simulink model "Sub1"  (R2024a)
settings: Solver=FixedStepDiscrete  StartTime=0.0  StopTime=1  FixedStep=7.5e-05  RelTol=1e-3  EnableMultiTasking=on
undefined symbols (not defined in the file or in its folder): D1, D11, Delta
libraries: spsSeriesRLCBranchLib x41, spsLoadFlowBusLib x29, spsDistributedParametersLineLib x19, spsThreePhaseSeriesRLCLoadLib x15, spsThreePhaseTransformerTwoWindingsLib x13, spsThreePhaseParallelRLCLoadLib x11, spsThreePhaseVIMeasurementLib x11, spsSynchronousMachinepuStandardLib x7, spsExcitationSystemLib x7, spsHydraulicTurbineandGovernorLib x7, spsGenericPowerSystemStabilizerLib x7, spsMultiBandPowerSystemStabilizerLib x7
(part 1 of 5)
settings Model: Creator=The MathWorks, Inc.  LastModifiedBy=dilu2
settings SolverCC: AlgebraicLoopSolver=TrustRegion
settings DataIOCC: SaveFormat=StructureWithTime  SaveOutput=off  SignalLogging=off  DSMLogging=off  SaveTime=off  ReturnWorkspaceOutputs=off
settings OptimizationCC: ExpressionDepthLimit=2147483647  LifeSpan=inf
settings DebuggingCC: UnderspecifiedInitializationDetection=Classic  MergeDetectMultiDrivingBlocksExec=none  SolverPrmCheckMsg=warning  FcnCallInpInsideContextMsg=warning  UnconnectedInputMsg=warning  UnconnectedOutputMsg=warning  UnconnectedLineMsg=warning  StateNameClashWarn=warning  SFUnexpectedBacktrackingDiag=warning  SFNoUnconditionalDefaultTransitionDiag=warning  SFExecutionAtInitializationDiag=none  ArithmeticOperatorsInVariantConditions=warning
settings HardwareCC: ProdBitPerPointer=32  ProdBitPerSizeT=32  ProdBitPerPtrDiffT=32  ProdLargestAtomicFloat=None  ProdIntDivRoundTo=Undefined  ProdEndianess=Unspecified  ProdWordSize=32  ProdHWDeviceType=32-bit Generic
settings ModelReferenceCC: EnableRefExpFcnMdlSchedulingChecks=on  PropagateSignalLabelsOutOfModel=off
settings SFSimCC: SimUseLocalCustomCode=off  CustomCodeUndefinedFunction=UseInterfaceOnly
settings RTWCC: RTWUseLocalCustomCode=off  GPUComputeCapability=3.5
settings CodeAppCC: StateflowObjectComments=on
settings GRTTargetCC: TargetLangStandard=C89/C90 (ANSI)  CombineOutputUpdateFcns=off  GRTInterface=on
settings ConfigComp: CovMetricSettings=dw  CovSaveCumulativeToWorkspaceVar=on  CovSaveSingleToWorkspaceVar=on  CovExternalEMLEnable=off  CovSFcnEnable=off
settings SimscapeCC: SimscapeNormalizeSystem=off

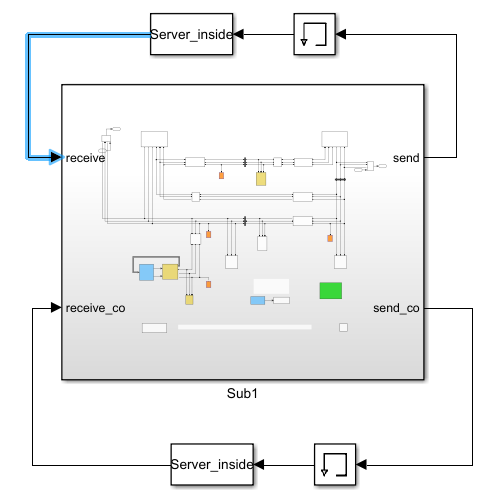
[thumbnail: Simulink's stored preview of the top-level diagram]
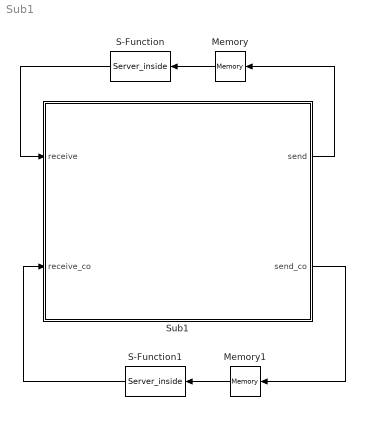
== system Sub1 ==
  Memory : Memory
  Memory1 : Memory
  S-Function : S-Function  FunctionName=Server_inside  SFunctionDeploymentMode=off  EnableBusSupport=off
  S-Function1 : S-Function  FunctionName=Server_inside  SFunctionDeploymentMode=off  EnableBusSupport=off
  Sub1 : Subsystem
  wires:
  Memory/1 -> S-Function/1
  Sub1/1(send) -> Memory/1
  S-Function/1 -> Sub1/1(receive)
  Memory1/1 -> S-Function1/1
  S-Function1/1 -> Sub1/2(receive_co)
  Sub1/2(send_co) -> Memory1/1

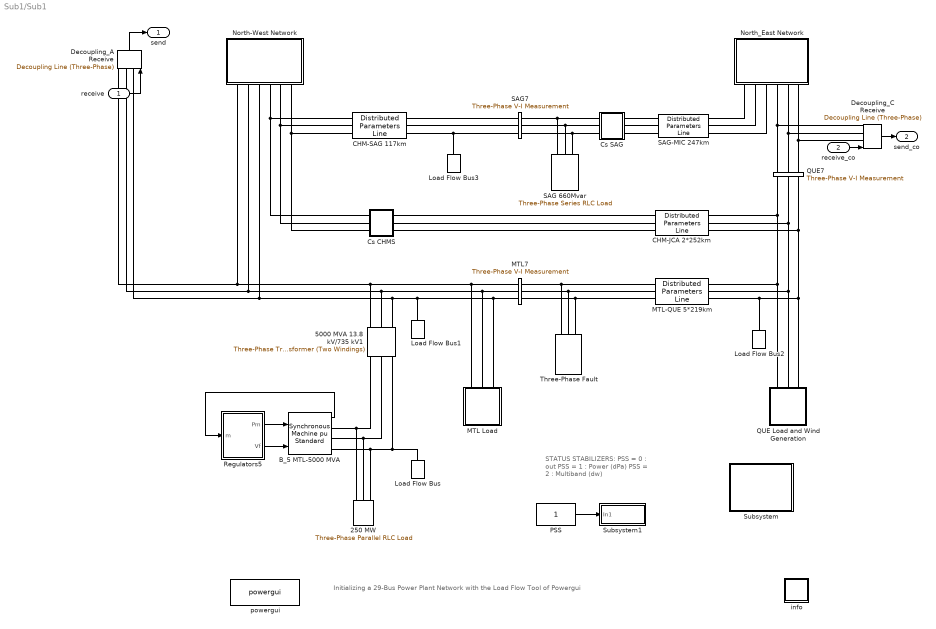
== system Sub1/Sub1 ==
  note: STATUS STABILIZERS:
      | PSS = 0 :  out
      | PSS = 1 :  Power (dPa)
      | PSS = 2 :  Multiband (dw)
  note: Initializing a 29-Bus Power Plant Network with the Load Flow Tool of Powergui
  receive : Inport
  receive_co : Inport  Port=2
  250 MW : spsThreePhaseParallelRLCLoadLib/Three-Phase Parallel RLC Load  LConnTagsString=A|B|C  Configuration=Y (grounded)  NominalVoltage=(13800)*1  Vabc=[1e3 1e3 1e3]  Vabcp=[1e3 1e3 1e3]  NominalFrequency=60  UnbalancedPower=off  ActivePower=250000000  InductivePower=0  CapacitivePower=0  Pabc=[10e3 9e3 11e3]  QLabc=[100 90 110]  QCabc=[100 90 110]  Pabcp=[10e3 9e3 11e3]  QLabcp=[100 90 110]  QCabcp=[100 90 110]  Measurements=None  LoadType=constant PQ
  5000 MVA 13.8 kV/735 kV1 : spsThreePhaseTransformerTwoWindingsLib/Three-Phase Transformer (Two Windings)  Winding1Connection=Delta (D1)  Winding2Connection=Yg  CoreType=Three single-phase transformers  SetSaturation=off  Hysteresis=off  DataFile='basic_model'  SetInitialFlux=off  Measurements=None  UNITS=pu  NominalPower=[ 5000e6 60 ]  Winding1="[ 13.8e3 0.002  0.0]"  Winding2=[ 735e3 0.002 0.12]  Rm=500  Lm=500  L0=0.5  Saturation="[ 0,0  ;  0.005,1.2  ;  1.0,1.4 ]"  InitialFluxes=[ 0.8 , -0.8 , 0.7 ]  BreakLoop=off  DiscreteSolver=Trapezoidal iterative  DataType=off  TransfoNumber=0
  B_5 MTL-5000 MVA : spsSynchronousMachinepuStandardLib/Synchronous Machine pu Standard  PresetModel=No  MechanicalLoad=Mechanical power Pm  ShowDetailedParameters=on  RotorType=Salient-pole  Units=per unit standard parameters  MeasurementBus=off  NominalParameters="[5000E6  13800   60 ]"  Reactances1=[ 31 32 33 34 35 36 37 ]  Reactances2=[ 1.305, 0.296, 0.252, 0.474, 0.243, 0.18 ]  dAxisTimeConstants=Short-circuit  qAxisTimeConstants=Open-circuit  TimeConstants1=[]  TimeConstants2=[]  TimeConstants3=[]  TimeConstants4=[]  TimeConstants5=[ 1.01, 0.053, 0.1 ]  TimeConstants6=[]  TimeConstants7=[]  TimeConstants8=[]  StatorResistance=2.8544e-3  Mechanical="[ 3.7 0  32]"  PolePairs=32  InitialConditions=[0 -113.876 0.904539 0.904539 0.904539 -42.1129 -162.113 77.8871 1.28555]  SetSaturation=off  Saturation=[0.6404,0.7127,0.8441,0.9214,0.9956,1.082,1.19,1.316,1.457;0.7,0.7698,0.8872,0.9466,0.9969,1.046,1.1,1.151,1.201]  LoadFlowParameters=[1 4000000000 0 0 0]  TsPowergui=0  TsBlock=-1  IterativeModel=Trapezoidal non iterative  IterativeDiscreteModel=Trapezoidal non iterative  BusType=PV  Pref=4500000000  Qref=0  Qmin=-Inf  Qmax=Inf  PLF=0  QLF=0
  CHM-JCA 2*252km : spsDistributedParametersLineLib/Distributed Parameters Line  Phases=3  Length=252  Frequency=60  Resistance="[0.01273  0.3864]/2"  Inductance="[0.9337e-3  4.1264e-3]/2"  Capacitance=[12.74e-9 7.751e-9]*2  x1=[-0.0015 2.14221721230477e-08 15714.2625948139 -742648.807936558;-0.001425 2.14666224013432e-08 36703.0761534274 -741907.71197206;-0.00135 2.14939125901414e-08 57662.5498345396 -740573.546334181;-0.001275 2.1504020874083e-08 78575.9289555807 -738647.377534517;-0.0012 2.14969391727604e-08 99426.4956812668 -736130.745322936;-0.001125 2.14726731471772e-08 120197.582387582 -733025.661456722;-0.00105 2.14312421952232e-08 140872.584985621 -729334.608092408;-0.000975 2.13726794361672e-08 161434.976194645 -725060.535801579;-0.0009 2.1297031684183e-08 181868.318753737 -720206.861212228;-0.000825 2.12043594109259e-08 202156.278561496 -714777.464277558;-0.00075 2.10947366971934e-08 222282.637733268 -708776.685174407;-0.000675 2.09682511737053e-08 242231.307565474 -702209.320833775;-0.0006 2.08250039510541e-08 261986.341396676 -695080.621106231;-0.000525 2.06651095388776e-08 281531.94735509 -687396.284565265;-0.00045 2.04886957543225e-08 300852.500982373 -679162.453951933;-0.000375 2.02959036198689e-08 319932.557723567 -670385.711264446;-0.0003 2.00868872505994e-08 338756.86527325 -661073.072496619;-0.000225 1.98618137310014e-08 357310.375767987 -651231.982029396;-0.00015 1.96208629814028e-08 375578.257815367 -640870.306679922;-7.5e-05 1.93642276141461e-08 393545.908349989 -629996.329412933]  x2=[-0.0015 1.38205484326445e-08 -209700.603633361 -700128.672634782;-0.001425 1.37920737733266e-08 -189823.746323616 -705777.196573591;-0.00135 1.37525739412601e-08 -169795.146815461 -710861.533020212;-0.001275 1.37020805120064e-08 -149630.815664894 -715377.617633884;-0.0012 1.36406338492402e-08 -129346.871929713 -719321.840325663;-0.001125 1.35682830724837e-08 -108959.530284185 -722691.048144279;-0.00105 1.34850860178407e-08 -88485.088057284 -725482.547796553;-0.000975 1.33911091917638e-08 -67939.9122048576 -727694.107800373;-0.0009 1.32864277178898e-08 -47340.4262261302 -729323.960268511;-0.000825 1.31711252769873e-08 -26703.0970350105 -730370.802321841;-0.00075 1.30452940400633e-08 -6044.42179669201 -730833.797130843;-0.000675 1.29090345946834e-08 14619.085259928 -730712.57458455;-0.0006 1.27624558645634e-08 35270.9060434707 -730007.231586412;-0.000525 1.26056750224974e-08 55894.5318043853 -728718.33197683;-0.00045 1.24388173966917e-08 76473.4763317904 -726846.906082429;-0.000375 1.22620163705793e-08 96991.2891322993 -724394.449892436;-0.0003 1.20754132761955e-08 117431.568580292 -721362.923862806;-0.000225 1.18791572811987e-08 137777.975029126 -717754.751349063;-0.00015 1.16734052696285e-08 158014.243872794 -713572.816669108;-7.5e-05 1.14583217164948e-08 178124.19854761 -708820.462797537]  x3=[-0.0015 5.44608144766307e-11 0.894999887860962 -284.908126309021;-0.001425 5.3877879205201e-11 8.94952227176843 -284.768519994184;-0.00135 5.32518747814939e-11 16.9968905445041 -284.401274081569;-0.001275 5.25833016238674e-11 25.0306717629996 -283.806682141938;-0.0012 5.18726941794743e-11 33.0444438454699 -282.98521948299;-0.001125 5.11206204970331e-11 41.0318007051272 -281.937542769407;-0.00105 5.03276817727381e-11 48.9863573711083 -280.664489497923;-0.000975 4.94945118696735e-11 56.9017550925234 -279.167077327845;-0.0009 4.86217768111116e-11 64.7716664215435 -277.446503267551;-0.000825 4.7710174248105e-11 72.589800271466 -275.504142717618;-0.00075 4.67604329017947e-11 80.3499069457126 -273.341548371352;-0.000675 4.57733119808813e-11 88.0457831337417 -270.960448973583;-0.0006 4.47496005747255e-11 95.6712768698793 -268.36274793874;-0.000525 4.36901170225622e-11 103.220292451107 -265.550521829281;-0.00045 4.25957082593322e-11 110.686795309872 -262.526018695731;-0.000375 4.14672491386559e-11 118.064816838032 -259.291656279619;-0.0003 4.03056417334883e-11 125.348459158063 -255.850020080773;-0.000225 3.9111814615016e-11 132.53189983774 -252.20386129051;-0.00015 3.78867221103713e-11 139.609396544492 -248.35609459238;-7.5e-05 3.66313435397578e-11 146.575291635741 -244.309795832209]  x4=[-0.0015 3.11331321468092e-11 -3172.83341993578 -10043.3125795458;-0.001425 3.24270107310813e-11 -2887.6355082528 -10128.9965094917;-0.00135 3.3694967659125e-11 -2600.12926492682 -10206.5834746068;-0.001275 3.49359893455722e-11 -2310.54451804977 -10276.0114530582;-0.0012 3.61490837366751e-11 -2019.11275723751 -10337.2249451823;-0.001125 3.73332811033385e-11 -1726.06694858057 -10390.17501785;-0.00105 3.84876348163062e-11 -1431.64134841465 -10434.8193435835;-0.000975 3.96112221028823e-11 -1136.07131605966 -10471.1222343919;-0.0009 4.07031447845814e-11 -839.593125677075 -10499.0546702996;-0.000825 4.17625299951187e-11 -542.443777396034 -10518.5943225447;-0.00075 4.2788530878166e-11 -244.860807859011 -10529.7255714284;-0.000675 4.37803272643159e-11 52.9178996613191 -10532.4395188004;-0.0006 4.4737126326712e-11 350.65430542233 -10526.7339951728;-0.000525 4.56581632148236e-11 648.110403496778 -10512.613561454;-0.00045 4.65427016658546e-11 945.048412031093 -10490.0895053025;-0.000375 4.73900345933011e-11 1241.23096332455 -10459.1798321041;-0.0003 4.81994846521856e-11 1536.42129357741 -10419.9092505789;-0.000225 4.8970404780516e-11 1830.38343215621 -10372.3091530287;-0.00015 4.97021787165371e-11 2122.88239022515 -10316.4175902431;-7.5e-05 5.03942214913611e-11 2413.68434859253 -10252.2792410825]  x5=0.00142516474882927  V1=ones(3,3)  V2=ones(3,3)  I1=ones(3,3)  I2=ones(3,3)  nHarmo=1  Measurements=None  Decoupling=on  VsMag0=[606505.937088368 606505.596193701 606505.952336057]  VrMag0=[596743.7373363 596743.911083318 596743.706580261]  VsAngle0=[3.61218308623452 -116.387796657607 123.612221103661]  VrAngle0=[-14.2738568821649 -134.273869923457 105.726122150019]  IsMag0=[234.023435046449 234.012623108521 234.010085804401]  IrMag0=[8650.90032066112 8650.90619032951 8650.91364627791]  IsAngle0=[2.58186505637036 -117.420380634471 122.583034804929]  IrAngle0=[-15.1321830152081 -135.132103549671 104.86782305054]
      settings: AttributesFormatString=\n  LibrarySourceBlock=sps_lib/Power Grid Elements/Distributed Parameters Line
  CHM-SAG 117km : spsDistributedParametersLineLib/Distributed Parameters Line  Phases=3  Length=117  Frequency=60  Resistance="[0.01273  0.3864]"  Inductance="[0.9337e-3  4.1264e-3]"  Capacitance=[12.74e-9 7.751e-9]  x1=[-0.000675 1.99891011372801e-08 161384.253868444 -730188.013920946;-0.0006 1.9861149341103e-08 181962.578167346 -725333.731757044;-0.000525 1.97173208460285e-08 202395.444365381 -719899.628905954;-0.00045 1.95577306263547e-08 222666.518741945 -713890.04930635;-0.000375 1.93825062560616e-08 242759.596910338 -707309.796924214;-0.0003 1.91917878068296e-08 262658.616771308 -700164.131912621;-0.000225 1.89857277360691e-08 282347.671352842 -692458.766406846;-0.00015 1.87644907650477e-08 301811.021525961 -684199.859958181;-7.5e-05 1.85282537472151e-08 321033.108586336 -675394.014610073]  x2=[-0.000675 1.35443395855415e-08 211241.020698681 -709610.35423456;-0.0006 1.3439585589586e-08 231217.67857916 -703354.834381312;-0.000525 1.33240881945427e-08 251009.504585131 -696537.063435149;-0.00045 1.31979397272621e-08 270600.677433712 -689162.49141785;-0.000375 1.30612410288988e-08 289975.536241081 -681237.013449452;-0.0003 1.29141013743006e-08 309118.593041554 -672766.965035778;-0.000225 1.27566383846562e-08 328014.545168422 -663759.117003934;-0.00015 1.25889779334703e-08 346648.287486673 -654220.670089812;-7.5e-05 1.24112540459421e-08 365004.924467804 -644159.249181932]  x3=[-0.000675 1.53428175208454e-11 931.801693491229 -3923.77003572275;-0.0006 1.4387032050888e-11 1042.3568642952 -3895.8590867212;-0.000525 1.34197458076381e-11 1152.07879097044 -3864.83384757437;-0.00045 1.24417320249186e-11 1260.87976348758 -3830.71911938373;-0.000375 1.14537725119832e-11 1368.67280801389 -3793.54217294102;-0.0003 1.04566570285503e-11 1475.37175643888 -3753.33272692841;-0.000225 9.45118265348109e-12 1580.89131525571 -3710.1229241618;-0.00015 8.43815314760658e-12 1685.14713374358 -3663.94730589641;-7.5e-05 7.41837831121395e-12 1788.05587139634 -3614.84278421495]  x4=[-0.000675 2.95936100054461e-11 34.7429415928699 -1477.32347167436;-0.0006 3.04376849592254e-11 76.4934319413223 -1475.75088744153;-0.000525 3.12574284933605e-11 118.18277461067 -1472.99861052903;-0.00045 3.20521853174128e-11 159.77764377825 -1469.06884106491;-0.000375 3.28213201149371e-11 201.244789142075 -1463.96472044674;-0.0003 3.35642180513446e-11 242.551062500607 -1457.69032883046;-0.000225 3.42802852653917e-11 283.663444250933 -1450.25068186873;-0.00015 3.49689493439035e-11 324.54906978412 -1441.65172670148;-7.5e-05 3.56296597793527e-11 365.175255756689 -1431.90033720193]  x5=0.000661683633385019  V1=ones(3,3)  V2=ones(3,3)  I1=ones(3,3)  I2=ones(3,3)  nHarmo=1  Measurements=None  Decoupling=on  VsMag0=[610584.183721697 610584.009535635 610584.144429957]  VrMag0=[604521.569069116 604521.776249676 604521.565003162]  VsAngle0=[-2.95698942544552 -122.956984245972 117.043027319658]  VrAngle0=[1.15752648646782 -118.842485295545 121.157503589919]  IsMag0=[3301.92473587883 3301.92030404023 3301.91445622762]  IrMag0=[1209.87683704235 1209.87940955581 1209.8866532217]  IsAngle0=[-2.06102029188666 -122.061181862044 117.938965522653]  IrAngle0=[-14.0730509971337 -134.072584557043 105.927076719811]
      settings: AttributesFormatString=\n  LibrarySourceBlock=sps_lib/Power Grid Elements/Distributed Parameters Line
  Cs CHMS : Subsystem  mask{Xc=33/2}
      mask prompts: Xc "Condensator Reactance at  60Hz  (ohm):"
      mask help: Series Compensation
      mask init:
      | Cs=1/Xc/(2*pi*60);
      mask Display: disp('Cs')
  Cs SAG : Subsystem  mask{Xc=22}
      mask prompts: Xc "Condensator Reactance at  60Hz  (ohm):"
      mask help: Series Compensation
      mask init:
      | Cs=1/Xc/(2*pi*60);
      mask Display: disp('Cs')
  Decoupling_A Receive : spsDecouplingLineThreePhaseLib/Decoupling Line (Three-Phase)  Length=252  Frequency=60  Resistance="[0.01273  0.3864]/2"  Inductance="[0.9337e-3  4.1264e-3]/2"  Capacitance=[12.74e-9 7.751e-9]*2  VsMag0=[520613.01336377 520613.032750475 520613.042981105]  VsAngle0=[95.9069967092304 -144.093005822699 -24.0930027089851]  IhsMag0=[3886.8321505435 3886.83229528581 3886.83237166039]  IhsAngle0=[86.4922430478116 -153.507759484046 -33.5077563703122]  ShowPorts=on  ConnectorID=T42_4042_2844522148740_R
      settings: LibrarySourceBlock=|
      | sps_lib/Power Grid Elements/Decoupling Line
      | (Three-Phase)
  Decoupling_C Receive : spsDecouplingLineThreePhaseLib/Decoupling Line (Three-Phase)  Length=252  Frequency=60  Resistance="[0.01273  0.3864]/2"  Inductance="[0.9337e-3  4.1264e-3]/2"  Capacitance=[12.74e-9 7.751e-9]*2  VsMag0=[539326.065002207 539326.156042215 539326.02070903]  VsAngle0=[103.825331452952 -136.17465752961 -16.1746546623784]  IhsMag0=[3629.74540447128 3629.74477875179 3629.75000907213]  IhsAngle0=[47.3040516013799 167.303961970658 -72.6960017677198]  ShowPorts=on  ConnectorID=T42_4044_2849153755848_R
      settings: LibrarySourceBlock=|
      | sps_lib/Power Grid Elements/Decoupling Line
      | (Three-Phase)
  Load Flow Bus : spsLoadFlowBusLib/Load Flow Bus  LConnTagsString=a  Phases=single  Connectors=on one side  ID=MTL_13.8  Vbase=13.8e3  Vref=1  Vangle=0  VLF=1  VLFb=1  VLFc=1  angleLF=-47.86  angleLFb=0  angleLFc=0
      settings: AttributesFormatString=%<ID>\n%<Vbase>V\n%<VLF>pu\n%<angleLF>deg.
  Load Flow Bus1 : spsLoadFlowBusLib/Load Flow Bus  LConnTagsString=a  Phases=single  Connectors=on one side  ID=MTL7  Vbase=735e3  Vref=1  Vangle=0  VLF=1.013  VLFb=1  VLFc=1  angleLF=-23.64  angleLFb=0  angleLFc=0
      settings: AttributesFormatString=%<ID>\n%<Vbase>V\n%<VLF>pu\n%<angleLF>deg.
  Load Flow Bus2 : spsLoadFlowBusLib/Load Flow Bus  LConnTagsString=a  Phases=single  Connectors=on one side  ID=QUE7  Vbase=735e3  Vref=1  Vangle=0  VLF=1.023  VLFb=1  VLFc=1  angleLF=-14.99  angleLFb=0  angleLFc=0
      settings: AttributesFormatString=%<ID>\n%<Vbase>V\n%<VLF>pu\n%<angleLF>deg.
  Load Flow Bus3 : spsLoadFlowBusLib/Load Flow Bus  LConnTagsString=a  Phases=single  Connectors=on one side  ID=SAG7  Vbase=735e3  Vref=1  Vangle=0  VLF=1.036  VLFb=1  VLFc=1  angleLF=-0.1653  angleLFb=0  angleLFc=0
      settings: AttributesFormatString=%<ID>\n%<Vbase>V\n%<VLF>pu\n%<angleLF>deg.
  MTL Load : Subsystem
  MTL-QUE 5*219km : spsDistributedParametersLineLib/Distributed Parameters Line  Phases=3  Length=219  Frequency=60  Resistance="[0.01273  0.3864]/5"  Inductance="[0.9337e-3  4.1264e-3]/5"  Capacitance=[12.74e-9 7.751e-9]*5  x1=[-0.001275 8.77181315970738e-08 0 0;-0.0012 8.77107360569241e-08 0 0;-0.001125 8.76332258963897e-08 0 0;-0.00105 8.74856630759072e-08 0 0;-0.000975 8.72681655549372e-08 0 0;-0.0009 8.69809071976704e-08 0 0;-0.000825 8.66241176340422e-08 -143097.879675145 -713663.77653496;-0.00075 8.61980820761709e-08 -122864.998636688 -717423.987747089;-0.000675 8.57031410903627e-08 -102533.901198218 -720610.701200368;-0.0006 8.51396903248689e-08 -82120.8397279515 -723221.369484821;-0.000525 8.45081801936104e-08 -61642.1321148977 -725253.905672165;-0.00045 8.38091155161236e-08 -41114.1487245874 -726706.684984072;-0.000375 8.30430551140157e-08 -20553.2993128542 -727578.546090988;-0.0003 8.2210611364251e-08 23.9800918736146 -727868.792040484;-0.000225 8.13124497096263e-08 20601.2403272829 -727577.190814389;-0.00015 8.03492881268259e-08 41162.0322463841 -726703.975514261;-7.5e-05 7.93218965524822e-08 61689.9198667078 -725249.844175051]  x2=[-0.001275 1.37020805120064e-08 0 0;-0.0012 1.36406338492402e-08 0 0;-0.001125 1.35682830724837e-08 0 0;-0.00105 1.34850860178407e-08 0 0;-0.000975 1.33911091917638e-08 0 0;-0.0009 1.32864277178898e-08 0 0;-0.000825 1.31711252769873e-08 -26703.0970350105 -730370.802321841;-0.00075 1.30452940400633e-08 -6044.42179669201 -730833.797130843;-0.000675 1.29090345946834e-08 14619.085259928 -730712.57458455;-0.0006 1.27624558645634e-08 35270.9060434707 -730007.231586412;-0.000525 1.26056750224974e-08 55894.5318043853 -728718.33197683;-0.00045 1.24388173966917e-08 76473.4763317904 -726846.906082429;-0.000375 1.22620163705793e-08 96991.2891322993 -724394.449892436;-0.0003 1.20754132761955e-08 117431.568580292 -721362.923862806;-0.000225 1.18791572811987e-08 137777.975029126 -717754.751349063;-0.00015 1.16734052696285e-08 158014.243872794 -713572.816669108;-7.5e-05 1.14583217164948e-08 178124.19854761 -708820.462797537]  x3=[-0.001275 3.4872588394047e-10 0 0;-0.0012 3.23593245705893e-10 0 0;-0.001125 2.98201931981841e-10 0 0;-0.00105 2.72572240196005e-10 0 0;-0.000975 2.46724658331852e-10 0 0;-0.0009 2.20679848550842e-10 0 0;-0.000825 1.94458630675415e-10 -5323.24056616586 -20344.1866352293;-0.00075 1.68081965545943e-10 -4745.97060123456 -20486.5462812041;-0.000675 1.41570938264955e-10 -4164.90678002043 -20612.5292955363;-0.0006 1.14946741342025e-10 -3580.51359605155 -20722.034969332;-0.000525 8.82306577528103e-11 -2993.25820429769 -20814.9757654309;-0.00045 6.14440439257625e-11 -2403.6100477337 -20891.2773883828;-0.000375 3.46083126701258e-11 -1812.04048207402 -20950.8788438376;-0.0003 7.74491605886562e-12 -1219.02239897811 -20993.7324873039;-0.000225 -1.91246717197908e-11 -625.029848028136 -21019.8040622347;-0.00015 -4.59789715284918e-11 -30.5376577809207 -21029.072727412;-7.5e-05 -7.27965164508547e-11 563.978943802682 -21021.5310736065]  x4=[-0.001275 2.87682179158487e-10 0 0;-0.0012 3.16443472016044e-10 0 0;-0.001125 3.44951804803819e-10 0 0;-0.00105 3.73184388396773e-10 0 0;-0.000975 4.01118654099555e-10 0 0;-0.0009 4.28732271687571e-10 0 0;-0.000825 4.56003167257424e-10 -1592.00824148586 -5672.40977475983;-0.00075 4.82909540872454e-10 -1431.01007071809 -5715.1495706848;-0.000675 5.09429883989274e-10 -1268.86797239497 -5753.32076348769;-0.0006 5.35542996651371e-10 -1105.71156042906 -5786.892839701;-0.000525 5.61228004436029e-10 -941.671259559694 -5815.83896232069;-0.00045 5.86464375141016e-10 -776.878201093489 -5840.13599225922;-0.000375 6.11231935197721e-10 -611.464118079965 -5859.76450684261;-0.0003 6.35510885797592e-10 -445.561240006162 -5874.70881533664;-0.000225 6.59281818718999e-10 -279.302187094414 -5884.95697148975;-0.00015 6.82525731841872e-10 -112.81986428777 -5890.5007830827;-7.5e-05 7.05224044337704e-10 53.7526449921845 -5891.33581847735]  x5=0.00123853603172068  V1=ones(3,3)  V2=ones(3,3)  I1=ones(3,3)  I2=ones(3,3)  nHarmo=1  Measurements=None  Decoupling=on  VsMag0=[594302.51828106 594302.52559147 594302.380387351]  VrMag0=[596743.7373363 596743.911083318 596743.706580261]  VsAngle0=[-23.5181046799956 -143.518120437643 96.4818868308235]  VrAngle0=[-14.2738568821649 -134.273869923457 105.726122150019]  IsMag0=[17258.8321886679 17258.8369567313 17258.8217052458]  IrMag0=[4835.28137561633 4835.2797345954 4835.28879561515]  IsAngle0=[-26.8431826212182 -146.843231946902 93.1567790076253]  IrAngle0=[-27.857296446876 -147.857183694833 92.1427767692303]
      settings: AttributesFormatString=\n  LibrarySourceBlock=sps_lib/Power Grid Elements/Distributed Parameters Line
  MTL7 : spsThreePhaseVIMeasurementLib/Three-Phase V-I Measurement  VoltageMeasurement=phase-to-ground  SetLabelV=on  LabelV=Vabc_MTL7  Vpu=on  VpuLL=off  CurrentMeasurement=no  SetLabelI=off  LabelI=A1  Ipu=off  Pbase=100e6  Vbase=735e3  OutputType=Magnitude  PhasorSimulation=off  PSBequivalent=0
  North-West Network : Subsystem
  North_East Network : Subsystem
  PSS : Constant
  QUE Load and Wind Generation : Subsystem
  QUE7 : spsThreePhaseVIMeasurementLib/Three-Phase V-I Measurement  VoltageMeasurement=no  SetLabelV=on  LabelV=Vabc_QUE7  Vpu=on  VpuLL=off  CurrentMeasurement=no  SetLabelI=off  LabelI=A1  Ipu=off  Pbase=100e6  Vbase=735e3  OutputType=Magnitude  PhasorSimulation=off  PSBequivalent=0
  Regulators5 : Subsystem
  SAG 660Mvar : spsThreePhaseSeriesRLCLoadLib/Three-Phase Series RLC Load  LConnTagsString=A|B|C  Configuration=Y (grounded)  NominalVoltage=735e3  Vabc=[1e3 1e3 1e3]  Vabcp=[1e3 1e3 1e3]  NominalFrequency=60  UnbalancedPower=off  ActivePower=2200000  InductivePower=660e6  CapacitivePower=0  Pabc=[10e3 9e3 11e3]  QLabc=[100 90 110]  QCabc=[100 90 110]  Pabcp=[10e3 9e3 11e3]  QLabcp=[100 90 110]  QCabcp=[100 90 110]  Measurements=None  LoadType=constant Z
  SAG-MIC 247km : spsDistributedParametersLineLib/Distributed Parameters Line  Phases=3  Length=247  Frequency=60  Resistance="[0.01273  0.3864]/1"  Inductance="[0.9337e-3  4.1264e-3]/1"  Capacitance=[12.74e-9 7.751e-9]*1  x1=[-0.001425 1.38793740392908e-08 -23892.3616667946 -729222.084146898;-0.00135 1.38614207140926e-08 -3267.28940141975 -729606.070163439;-0.001275 1.38323867812624e-08 17360.3946851114 -729406.820250838;-0.0012 1.37922954500819e-08 37974.2011377541 -728624.493686427;-0.001125 1.37411787689478e-08 58557.6515950321 -727259.715850092;-0.00105 1.36790775997528e-08 79094.2919615872 -725313.577724353;-0.000975 1.36060415852216e-08 99567.7055613315 -722787.635022251;-0.0009 1.35221291092265e-08 119961.526260687 -719683.906943734;-0.000825 1.3427407250117e-08 140259.451551422 -716004.874561539;-0.00075 1.3321951727098e-08 160445.255582629 -711753.478837862;-0.000675 1.3205846839701e-08 180502.802131418 -706933.118273395;-0.0006 1.30791854003967e-08 200416.057501969 -701547.64619062;-0.000525 1.29420686604015e-08 220169.103342621 -695601.367653519;-0.00045 1.27946062287394e-08 239746.149370761 -689099.036026173;-0.000375 1.26369159846222e-08 259131.545995333 -682045.849172997;-0.0003 1.24691239832181e-08 278309.796826883 -674447.445303644;-0.000225 1.22913643548859e-08 297265.571065131 -666309.898465907;-0.00015 1.21037791979525e-08 315983.715754186 -657639.713690219;-7.5e-05 1.19065184651223e-08 334449.26789558 -648443.821789632]  x2=[-0.001425 4.83884558825768e-09 88893.3544413917 -739233.912944048;-0.00135 4.81304910631898e-09 109756.40330769 -736425.413361802;-0.001275 4.78340514656681e-09 130531.714584513 -733028.226571802;-0.0012 4.74993740592903e-09 151202.6808059 -729045.068233188;-0.001125 4.71267263800543e-09 171752.777917729 -724479.122421791;-0.00105 4.67164063168132e-09 192165.578486796 -719334.039084833;-0.000975 4.62687418731474e-09 212424.764832653 -713613.931123211;-0.0009 4.57840909051637e-09 232514.142071711 -707323.371103708;-0.000825 4.52628408354304e-09 252417.651063182 -700467.387603755;-0.00075 4.47054083432781e-09 272119.381246513 -693051.461191662;-0.000675 4.41122390317118e-09 291603.583360041 -685081.520045535;-0.0006 4.34838070712034e-09 310854.682030716 -676563.935214383;-0.000525 4.28206148206469e-09 329857.288224812 -667505.515525196;-0.00045 4.21231924257801e-09 348596.211549686 -657913.502140075;-0.000375 4.13920973953947e-09 367056.472396749 -647795.562767757;-0.0003 4.06279141556716e-09 385223.31391593 -637159.785534167;-0.000225 3.98312535830005e-09 403082.213812081 -626014.672516893;-0.00015 3.90027525156537e-09 420618.895953875 -614369.132948754;-7.5e-05 3.8143073244708e-09 437819.341785928 -602232.476095899]  x3=[-0.001425 1.2965985215533e-11 -591.222973545921 -3970.47337116281;-0.00135 1.24748314580027e-11 -478.738749485255 -3985.60043687552;-0.001275 1.19737055110762e-11 -365.871828993199 -3997.54147458074;-0.0012 1.1463007967168e-11 -252.712436159072 -4006.2869387956;-0.001125 1.09431470700807e-11 -139.35102887011 -4011.82983852984;-0.00105 1.04145383886614e-11 -25.8782265008115 -4014.16574287422;-0.000975 9.87760448460195e-12 87.6152625268023 -4013.29278454253;-0.0009 9.33277457464995e-12 201.03871325411 -4009.21166136432;-0.000825 8.7804841874992e-12 314.301456710038 -4001.92563572701;-0.00075 8.22117481563489e-12 427.312952390445 -3991.44053196802;-0.000675 7.65529356241115e-12 539.98286063482 -3977.76473171886;-0.0006 7.08329278464353e-12 652.221114842417 -3960.90916720501;-0.000525 6.50562973100189e-12 763.937993470127 -3940.88731250683;-0.00045 5.92276617649276e-12 875.044191754501 -3917.71517278864;-0.000375 5.33516805332349e-12 985.45089310061 -3891.41127150436;-0.0003 4.74330507844322e-12 1095.06984008068 -3861.99663559024;-0.000225 4.14765037805823e-12 1203.81340498572 -3829.49477865616;-0.00015 3.5486801094222e-12 1311.59465987378 -3793.93168218925;-7.5e-05 2.94687308020333e-12 1418.3274460588 -3755.33577478471]  x4=[-0.001425 1.12481853077134e-11 -44.2696955265252 -1445.03567527874;-0.00135 1.18746078644322e-11 -3.40032222042646 -1445.70991618264;-0.001275 1.24915380413118e-11 37.4717692512286 -1445.22847869965;-0.0012 1.30984826738081e-11 78.3139063638814 -1443.59174768352;-0.001125 1.36949565796685e-11 119.09344053803 -1440.80103151198;-0.00105 1.42804829467789e-11 159.777773238003 -1436.85856104085;-0.000975 1.48545937143204e-11 200.334382030732 -1431.7674878207;-0.0009 1.54168299469296e-11 240.730846583684 -1425.53188157756;-0.000825 1.59667422015646e-11 280.934874581182 -1418.15672695966;-0.00075 1.6503890886783e-11 320.914327538389 -1409.64791955275;-0.000675 1.70278466141446e-11 360.637246492314 -1400.01226116729;-0.0006 1.75381905414575e-11 400.071877549329 -1389.25745440116;-0.000525 1.8034514707595e-11 439.186697268736 -1377.39209648233;-0.00045 1.85164223586125e-11 477.950437862128 -1364.42567239638;-0.000375 1.89835282649073e-11 516.33211218838 -1350.36854730432;-0.0003 1.94354590291649e-11 554.301038524295 -1335.23195825689;-0.000225 1.9871853384847e-11 591.826865091103 -1319.02800521175;-0.00015 2.02923624849829e-11 628.879594317213 -1301.76964136106;-7.5e-05 2.06966501810318e-11 665.429606817806 -1283.4706627768]  x5=0.00139688767047948  V1=ones(3,3)  V2=ones(3,3)  I1=ones(3,3)  I2=ones(3,3)  nHarmo=1  Measurements=None  Decoupling=on  VsMag0=[595726.858585719 595726.856922593 595726.834929636]  VrMag0=[607930.231676096 607930.976808471 607930.152146782]  VsAngle0=[-1.09657636563807 -121.096578900457 118.903422505479]  VrAngle0=[7.63692875075284 -112.363120449628 127.636843332424]  IsMag0=[3296.72064632885 3296.71771518482 3296.71033953515]  IrMag0=[1187.28543067548 1187.29227239652 1187.29553954431]  IsAngle0=[-7.68926033426529 -127.689437762275 112.310695069142]  IrAngle0=[-0.975042579697629 -120.974669903324 119.024857828981]
      settings: AttributesFormatString=\n  LibrarySourceBlock=sps_lib/Power Grid Elements/Distributed Parameters Line
  SAG7 : spsThreePhaseVIMeasurementLib/Three-Phase V-I Measurement  VoltageMeasurement=no  SetLabelV=on  LabelV=Vabc_SAG7  Vpu=on  VpuLL=off  CurrentMeasurement=no  SetLabelI=off  LabelI=Iabc_SAG7  Ipu=off  Pbase=100e6  Vbase=735e3  OutputType=Magnitude  PhasorSimulation=off  PSBequivalent=0
  Subsystem : Subsystem
      mask Display: disp('Display\nWaveforms')
  Subsystem1 : Subsystem
      mask Display: disp('PSS_select')
  Three-Phase Fault : spsThreePhaseFaultLib/Three-Phase Fault  InitialStates=0  FaultA=on  FaultB=on  FaultC=on  GroundFault=on  SwitchTimes=[0.2 0.3]  External=off  SwitchStatus=NaN  FaultResistance=0.001  GroundResistance=0.001  SnubberResistance=1e6  SnubberCapacitance=inf  Measurements=None
  info : Subsystem
      settings: OpenFcn="showExample(\"simscapeelectricalsps/LoadFlow29BusNetworkExample\")"
      mask Display: disp('?')
  powergui : sps_lib/powergui  Priority=1  SimulationMode=Discrete  SampleTime=75e-6  frequency=60  Iterations=50  frequencyindice=60  Pbase=1e+008  ErrMax=0.0001  UnitsV=kV  UnitsW=MW  buscounter=0  FunctionMessages=off  echomessages=off  EnableUseOfTLC=off  CurrentSourceSwitches=off  DisableSnubberDevices=off  DisableRonSwitches=off  DisableVfSwitches=off  DisplayEquations=off  AutomaticDiscreteSolvers=off  SolverType=Tustin/Backward Euler (TBE)  Interpol=off  ExternalGateDelay=off  methode=off  Ts=100  x0status=blocks  SPID=off  SwTol=0  HookPort=off  NonlinearTolerance=1e-4  nMaxIteration=100  ContinueOnMaxIteration=off  RestoreLinks=warning  ResistiveCurrentMeasurement=off  Frange=[0:2:500]  Ylog=off  Xlog=on  ShowGrid=off  save=off  variable=ZData  structure=0  ZoomFFT=off  StartTime=0.0  cycles=1  DisplayStyle=1  fundamental=60  FreqAxis=off  MaxFrequency=1000  frequencyindicesteady=1  RmsSteady=1  display=off
  send : Outport
  send_co : Outport  Port=2
  wires:
  receive/1 -> Decoupling_A Receive/1
  B_5 MTL-5000 MVA/1 -> Regulators5/1(m)
  Regulators5/1(Pm) -> B_5 MTL-5000 MVA/1
  Regulators5/2(Vf) -> B_5 MTL-5000 MVA/2
  PSS/1 -> Subsystem1/1(In1)
  Decoupling_A Receive/1 -> send/1
  Decoupling_C Receive/1 -> send_co/1
  receive_co/1 -> Decoupling_C Receive/1
  connections:
  MTL7/LConn2 -- MTL Load/LConn2 -- Decoupling_A Receive/LConn2 -- North-West Network/RConn2 -- 5000 MVA 13.8 kV/735 kV1/RConn2
  MTL7/LConn3 -- MTL Load/LConn3 -- Decoupling_A Receive/LConn1 -- North-West Network/RConn3 -- 5000 MVA 13.8 kV/735 kV1/RConn3 -- Load Flow Bus1/LConn1
  SAG-MIC 247km/RConn1 -- North_East Network/LConn1
  QUE Load and Wind Generation/LConn2 -- QUE7/LConn2 -- CHM-JCA 2*252km/RConn2 -- MTL-QUE 5*219km/RConn2
  250 MW/LConn2 -- 5000 MVA 13.8 kV/735 kV1/LConn2 -- B_5 MTL-5000 MVA/RConn2
  Load Flow Bus3/LConn1 -- CHM-SAG 117km/RConn3 -- SAG7/LConn3
  Cs CHMS/RConn3 -- CHM-JCA 2*252km/LConn3
  MTL7/LConn1 -- MTL Load/LConn1 -- Decoupling_A Receive/LConn3 -- North-West Network/RConn1 -- 5000 MVA 13.8 kV/735 kV1/RConn1
  QUE Load and Wind Generation/LConn1 -- MTL-QUE 5*219km/RConn1 -- QUE7/LConn1 -- CHM-JCA 2*252km/RConn1
  250 MW/LConn1 -- 5000 MVA 13.8 kV/735 kV1/LConn1 -- B_5 MTL-5000 MVA/RConn1
  Cs CHMS/LConn3 -- CHM-SAG 117km/LConn3 -- North-West Network/RConn6
  Cs CHMS/RConn1 -- CHM-JCA 2*252km/LConn1
  Cs SAG/LConn1 -- SAG7/RConn1 -- SAG 660Mvar/LConn1
  Cs SAG/RConn3 -- SAG-MIC 247km/LConn3
  Cs SAG/RConn2 -- SAG-MIC 247km/LConn2
  Cs SAG/LConn3 -- SAG7/RConn3 -- SAG 660Mvar/LConn3
  Cs CHMS/LConn2 -- CHM-SAG 117km/LConn2 -- North-West Network/RConn5
  QUE7/RConn3 -- North_East Network/LConn6 -- Decoupling_C Receive/LConn1
  QUE Load and Wind Generation/LConn3 -- QUE7/LConn3 -- CHM-JCA 2*252km/RConn3 -- MTL-QUE 5*219km/RConn3 -- Load Flow Bus2/LConn1
  MTL7/RConn3 -- Three-Phase Fault/LConn3 -- MTL-QUE 5*219km/LConn3
  MTL7/RConn1 -- Three-Phase Fault/LConn1 -- MTL-QUE 5*219km/LConn1
  Cs SAG/RConn1 -- SAG-MIC 247km/LConn1
  Cs CHMS/LConn1 -- CHM-SAG 117km/LConn1 -- North-West Network/RConn4
  QUE7/RConn1 -- Decoupling_C Receive/LConn3 -- North_East Network/LConn4
  QUE7/RConn2 -- Decoupling_C Receive/LConn2 -- North_East Network/LConn5
  Cs SAG/LConn2 -- SAG7/RConn2 -- SAG 660Mvar/LConn2
  5000 MVA 13.8 kV/735 kV1/LConn3 -- Load Flow Bus/LConn1 -- 250 MW/LConn3 -- B_5 MTL-5000 MVA/RConn3
  SAG7/LConn1 -- CHM-SAG 117km/RConn1
  SAG-MIC 247km/RConn2 -- North_East Network/LConn2
  Cs CHMS/RConn2 -- CHM-JCA 2*252km/LConn2
  MTL7/RConn2 -- Three-Phase Fault/LConn2 -- MTL-QUE 5*219km/LConn2
  SAG-MIC 247km/RConn3 -- North_East Network/LConn3
  SAG7/LConn2 -- CHM-SAG 117km/RConn2

== system Sub1/Sub1/Cs CHMS ==
  note: B
  Ca : spsSeriesRLCBranchLib/Series RLC Branch  LConnTagsString=__new0  RConnTagsString=__new0  BranchType=C  Resistance=1.0  Inductance=1.0  SetiL0=off  InitialCurrent=0  Capacitance=Cs  Setx0=off  InitialVoltage=0  Measurements=None
  Cb : spsSeriesRLCBranchLib/Series RLC Branch  LConnTagsString=__new0  RConnTagsString=__new0  BranchType=C  Resistance=1.0  Inductance=1.0  SetiL0=off  InitialCurrent=0  Capacitance=Cs  Setx0=off  InitialVoltage=0  Measurements=None
  Cc : spsSeriesRLCBranchLib/Series RLC Branch  LConnTagsString=__new0  RConnTagsString=__new0  BranchType=C  Resistance=1.0  Inductance=1.0  SetiL0=off  InitialCurrent=0  Capacitance=Cs  Setx0=off  InitialVoltage=0  Measurements=None
  A : PMIOPort  Side=Left
  B : PMIOPort  Port=2  Side=Left
  C : PMIOPort  Port=3  Side=Left
  "A " : PMIOPort  Port=4  Side=Right
  "B " : PMIOPort  Port=5  Side=Right
  "C " : PMIOPort  Port=6  Side=Right
  connections:
  Cc/RConn1 -- "C "/RConn1
  C/RConn1 -- Cc/LConn1
  Cb/RConn1 -- "B "/RConn1
  B/RConn1 -- Cb/LConn1
  Ca/RConn1 -- "A "/RConn1
  A/RConn1 -- Ca/LConn1

== system Sub1/Sub1/Cs SAG ==
  note: B
  Ca : spsSeriesRLCBranchLib/Series RLC Branch  LConnTagsString=__new0  RConnTagsString=__new0  BranchType=C  Resistance=1.0  Inductance=1.0  SetiL0=off  InitialCurrent=0  Capacitance=Cs  Setx0=off  InitialVoltage=0  Measurements=None
  Cb : spsSeriesRLCBranchLib/Series RLC Branch  LConnTagsString=__new0  RConnTagsString=__new0  BranchType=C  Resistance=1.0  Inductance=1.0  SetiL0=off  InitialCurrent=0  Capacitance=Cs  Setx0=off  InitialVoltage=0  Measurements=None
  Cc : spsSeriesRLCBranchLib/Series RLC Branch  LConnTagsString=__new0  RConnTagsString=__new0  BranchType=C  Resistance=1.0  Inductance=1.0  SetiL0=off  InitialCurrent=0  Capacitance=Cs  Setx0=off  InitialVoltage=0  Measurements=None
  A : PMIOPort  Side=Left
  B : PMIOPort  Port=2  Side=Left
  C : PMIOPort  Port=3  Side=Left
  "A " : PMIOPort  Port=4  Side=Right
  "B " : PMIOPort  Port=5  Side=Right
  "C " : PMIOPort  Port=6  Side=Right
  connections:
  A/RConn1 -- Ca/LConn1
  Ca/RConn1 -- "A "/RConn1
  B/RConn1 -- Cb/LConn1
  Cb/RConn1 -- "B "/RConn1
  C/RConn1 -- Cc/LConn1
  Cc/RConn1 -- "C "/RConn1

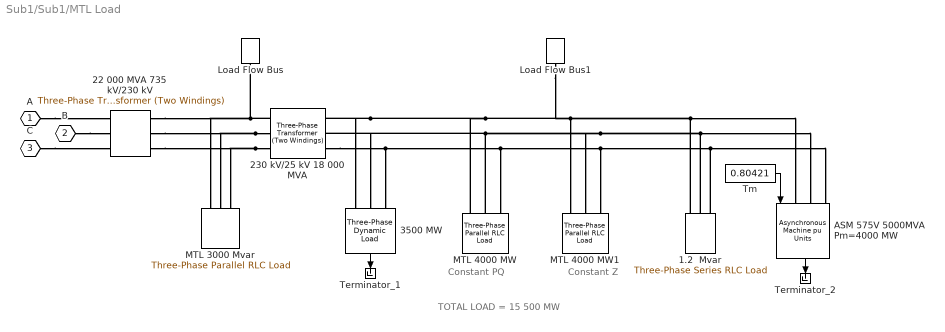
== system Sub1/Sub1/MTL Load ==
  note: Constant PQ
  note: Constant Z
  note: TOTAL LOAD = 15 500 MW
  1.2  Mvar : spsThreePhaseSeriesRLCLoadLib/Three-Phase Series RLC Load  LConnTagsString=A|B|C  Configuration=Y (grounded)  NominalVoltage=25e3  Vabc=[1e3 1e3 1e3]  Vabcp=[1e3 1e3 1e3]  NominalFrequency=60  UnbalancedPower=off  ActivePower=2000e6/50  InductivePower=0  CapacitivePower=2000e6  Pabc=[10e3 9e3 11e3]  QLabc=[100 90 110]  QCabc=[100 90 110]  Pabcp=[10e3 9e3 11e3]  QLabcp=[100 90 110]  QCabcp=[100 90 110]  Measurements=None  LoadType=constant Z
  22 000 MVA 735 kV/230 kV : spsThreePhaseTransformerTwoWindingsLib/Three-Phase Transformer (Two Windings)  Winding1Connection=Yg  Winding2Connection=Delta (D1)  CoreType=Three single-phase transformers  SetSaturation=off  Hysteresis=off  DataFile='basic_model'  SetInitialFlux=off  Measurements=None  UNITS=pu  NominalPower=[ 22000e6 60 ]  Winding1="[ 735e3 0.002  0.12]"  Winding2=[230e3 0.002 0]  Rm=500  Lm=500  L0=0.5  Saturation="[ 0,0  ;  0.005,1.2  ;  1.0,1.4 ]"  InitialFluxes=[ 0.8 , -0.8 , 0.7 ]  BreakLoop=off  DiscreteSolver=Trapezoidal iterative  DataType=off  TransfoNumber=0
  230 kV/25 kV 18 000 MVA : spsThreePhaseTransformerTwoWindingsLib/Three-Phase Transformer (Two Windings)  Winding1Connection=Yg  Winding2Connection=Delta (D1)  CoreType=Three single-phase transformers  SetSaturation=off  Hysteresis=off  DataFile='basic_model'  SetInitialFlux=off  Measurements=None  UNITS=pu  NominalPower=[18000e6 60 ]  Winding1="[ 230e3  0.08/30   0.08 ]"  Winding2="[ 25e3  0.08/30  0.08]"  Rm=500  Lm=500  L0=0.5  Saturation="[ 0,0  ;  0.005,1.2  ;  1.0,1.4 ]"  InitialFluxes=[ 0.8 , -0.8 , 0.7 ]  BreakLoop=off  DiscreteSolver=Trapezoidal iterative  DataType=off  TransfoNumber=0
  3500 MW : spsThreePhaseDynamicLoadLib/Three-Phase Dynamic Load  NominalVoltage=[ 25e3 60 ]  ActiveReactivePowers=[3.5e+09 4.44089e-08]  PositiveSequence=[0.991615 -96.3945]  ExternalControl=off  NpNq="[1.5  2.5]"  TimeConstants="[0  0  0  0]"  MinimumVoltage=0.7  Tfilter=1e-4  LoadFlowParameters=[4,0,0,0,0]
      settings: LibrarySourceBlock=|
      | sps_lib/Passives/Three-Phase
      | Dynamic Load
  ASM 575V 5000MVA Pm=4000 MW : spsAsynchronousMachinepuUnitsLib/Asynchronous Machine pu Units  RotorType=Squirrel-cage  PresetModel=No  MechanicalLoad=Torque Tm  ShowDetailedParameters=on  ReferenceFrame=Rotor  Units=pu  MeasurementBus=off  NominalParameters="[5000e6 25e3  60]"  VoltageRatio=1  Stator=[0.01117 0.04832]  Rotor=[0.006 0.04832]  Cage1=[0.01909 0.0397]  Cage2=[0.01909 0.0397]  Lm=2.424  Mechanical="[1  0   2]"  PolePairs=2  InitialConditions=[0.00523668 0 0.941796 0.941796 0.941796 -125.733 -245.733 -5.73298]  SimulateSaturation=off  Saturation="[0.212,0.4201,0.8125,1.0979,1.4799,2.2457,3.2586,4.5763,6.4763 ;   0.5,0.7,0.9,1,1.1,1.2 ,1.3,1.4,1.5]"  LoadFlowParameters=0  TsPowergui=0  TsBlock=-1  IterativeModel=Trapezoidal non iterative  IterativeDiscreteModel=Trapezoidal non iterative  Pmec=4000000000
      settings: LibrarySourceBlock=|
      | sps_lib/Electrical Machines/Asynchronous Machine
      | pu Units
  Load Flow Bus : spsLoadFlowBusLib/Load Flow Bus  LConnTagsString=a  Phases=single  Connectors=on one side  ID=MTL2  Vbase=230e3  Vref=1  Vangle=0  VLF=1.009  VLFb=1  VLFc=1  angleLF=-58.45  angleLFb=0  angleLFc=0
      settings: AttributesFormatString=%<ID>\n%<Vbase>V\n%<VLF>pu\n%<angleLF>deg.
  Load Flow Bus1 : spsLoadFlowBusLib/Load Flow Bus  LConnTagsString=a  Phases=single  Connectors=on one side  ID=MTL_25  Vbase=25e3  Vref=1  Vangle=0  VLF=0.9916  VLFb=1  VLFc=1  angleLF=-96.39  angleLFb=0  angleLFc=0
      settings: AttributesFormatString=%<ID>\n%<Vbase>V\n%<VLF>pu\n%<angleLF>deg.
  MTL 3000 Mvar : spsThreePhaseParallelRLCLoadLib/Three-Phase Parallel RLC Load  LConnTagsString=A|B|C  Configuration=Y (grounded)  NominalVoltage=230e3  Vabc=[1e3 1e3 1e3]  Vabcp=[1e3 1e3 1e3]  NominalFrequency=60  UnbalancedPower=off  ActivePower=0  InductivePower=0  CapacitivePower=3000e6  Pabc=[10e3 9e3 11e3]  QLabc=[100 90 110]  QCabc=[100 90 110]  Pabcp=[10e3 9e3 11e3]  QLabcp=[100 90 110]  QCabcp=[100 90 110]  Measurements=None  LoadType=constant Z
  MTL 4000 MW : spsThreePhaseParallelRLCLoadLib/Three-Phase Parallel RLC Load  LConnTagsString=A|B|C  Configuration=Y (grounded)  NominalVoltage=(25000)*0.991615  Vabc=[1e3 1e3 1e3]  Vabcp=[1e3 1e3 1e3]  NominalFrequency=60  UnbalancedPower=off  ActivePower=4000000000  InductivePower=0  CapacitivePower=0  Pabc=[10e3 9e3 11e3]  QLabc=[100 90 110]  QCabc=[100 90 110]  Pabcp=[10e3 9e3 11e3]  QLabcp=[100 90 110]  QCabcp=[100 90 110]  Measurements=None  LoadType=constant PQ
  MTL 4000 MW1 : spsThreePhaseParallelRLCLoadLib/Three-Phase Parallel RLC Load  LConnTagsString=A|B|C  Configuration=Y (grounded)  NominalVoltage=25e3  Vabc=[1e3 1e3 1e3]  Vabcp=[1e3 1e3 1e3]  NominalFrequency=60  UnbalancedPower=off  ActivePower=4000000000  InductivePower=0  CapacitivePower=0  Pabc=[10e3 9e3 11e3]  QLabc=[100 90 110]  QCabc=[100 90 110]  Pabcp=[10e3 9e3 11e3]  QLabcp=[100 90 110]  QCabcp=[100 90 110]  Measurements=None  LoadType=constant Z
  Terminator_1 : Terminator
  Terminator_2 : Terminator
  Tm : Constant  Value=0.80421
  A : PMIOPort  Side=Left
  B : PMIOPort  Port=2  Side=Left
  C : PMIOPort  Port=3  Side=Left
  wires:
  Tm/1 -> ASM 575V 5000MVA Pm=4000 MW/1
  3500 MW/1 -> Terminator_1/1
  ASM 575V 5000MVA Pm=4000 MW/1 -> Terminator_2/1
  connections:
  A/RConn1 -- 22 000 MVA 735 kV/230 kV/LConn1
  B/RConn1 -- 22 000 MVA 735 kV/230 kV/LConn2
  C/RConn1 -- 22 000 MVA 735 kV/230 kV/LConn3
  230 kV/25 kV 18 000 MVA/LConn1 -- Load Flow Bus/LConn1 -- 22 000 MVA 735 kV/230 kV/RConn1 -- MTL 3000 Mvar/LConn1
  230 kV/25 kV 18 000 MVA/LConn2 -- 22 000 MVA 735 kV/230 kV/RConn2 -- MTL 3000 Mvar/LConn2
  230 kV/25 kV 18 000 MVA/LConn3 -- 22 000 MVA 735 kV/230 kV/RConn3 -- MTL 3000 Mvar/LConn3
  MTL 4000 MW1/LConn1 -- Load Flow Bus1/LConn1 -- MTL 4000 MW/LConn1 -- 230 kV/25 kV 18 000 MVA/RConn1 -- 3500 MW/LConn1 -- ASM 575V 5000MVA Pm=4000 MW/LConn1 -- 1.2  Mvar/LConn1
  MTL 4000 MW1/LConn2 -- MTL 4000 MW/LConn2 -- 230 kV/25 kV 18 000 MVA/RConn2 -- 3500 MW/LConn2 -- ASM 575V 5000MVA Pm=4000 MW/LConn2 -- 1.2  Mvar/LConn2
  230 kV/25 kV 18 000 MVA/RConn3 -- ASM 575V 5000MVA Pm=4000 MW/LConn3 -- 1.2  Mvar/LConn3 -- MTL 4000 MW1/LConn3 -- MTL 4000 MW/LConn3 -- 3500 MW/LConn3
